simulink model "sys"  (R2021a)
settings: Solver=VariableStepAuto  StartTime=0.0  StopTime=10.0  RelTol=1e-3
settings Model: Creator=Suman  LastModifiedBy=Suman

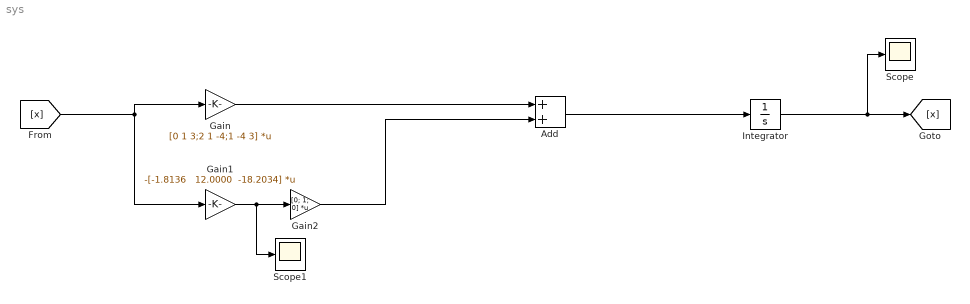
== system sys ==
  Add : Sum
  Gain : Gain  Gain=[0 1 3;2 1 -4;1 -4 3]  Multiplication=Matrix(K*u) (u vector)
  Gain1 : Gain  Gain="-[-1.8136   12.0000  -18.2034]"  Multiplication=Matrix(K*u) (u vector)
  Gain2 : Gain  Gain=[0; 1; 0]  Multiplication=Matrix(K*u)
  Integrator : Integrator  InitialCondition=[2;3;1]
  Scope : Scope
  Scope1 : Scope
  wires:
  Add/1 -> Integrator/1
  [x] -> Gain1/1, Gain/1
  Integrator/1 -> Scope/1, [x]
  Gain1/1 -> Scope1/1, Gain2/1
  Gain/1 -> Add/1
  Gain2/1 -> Add/2
